simulink model "posture_regulation"  (R2022b)
settings: Solver=VariableStepAuto  StartTime=0.0  StopTime=20  RelTol=1e-3
model workspace (MAT data in the model file):
  initial_conditions = [0 0 0]
values from neighbouring files (symbols this model uses):
  initial_conditions_trans = state_transformation([0,0,0], initial_conditions)    [init.m]
settings Model: Creator=dipietrant  LastModifiedBy=Edp
settings SolverCC: AlgebraicLoopSolver=TrustRegion
settings DebuggingCC: UnconnectedInputMsg=warning  UnconnectedOutputMsg=warning  UnconnectedLineMsg=warning  SFMachineParentedDataDiag=warning
settings ModelReferenceCC: EnableRefExpFcnMdlSchedulingChecks=on
settings RTWCC: DLArmComputeVersion=19.05

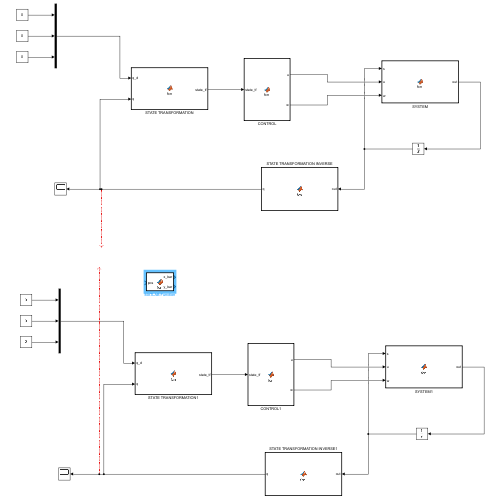
[thumbnail: Simulink's stored preview of the top-level diagram]
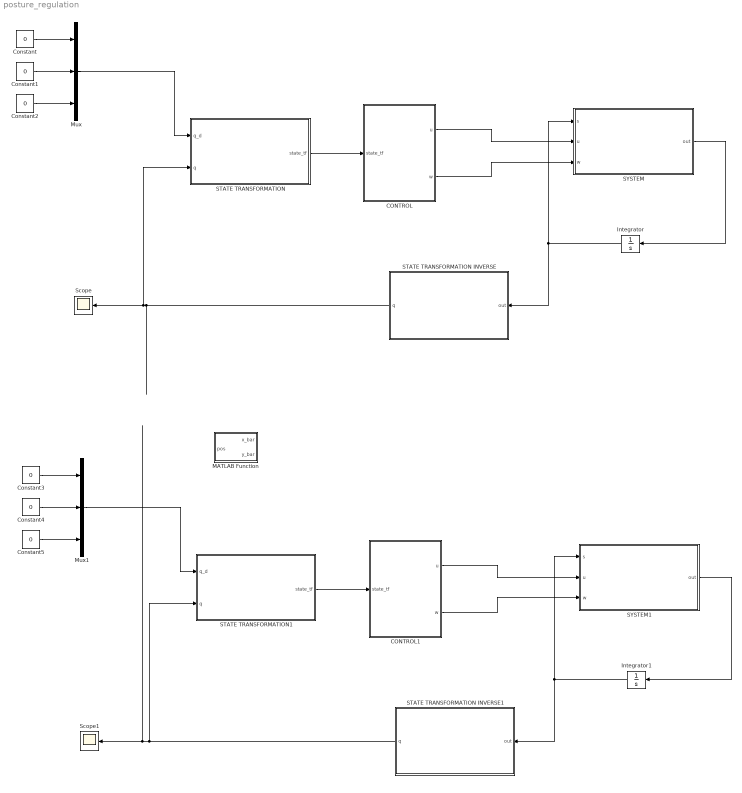
== system posture_regulation ==
  CONTROL : MATLAB Function  TreatAsAtomicUnit=on
  CONTROL1 : MATLAB Function  TreatAsAtomicUnit=on
  Constant{,1..5} (6 alike) : Constant  Value=0
  Integrator : Integrator  InitialCondition=initial_conditions_trans
  Integrator1 : Integrator  InitialCondition=initial_conditions_trans
  MATLAB Function : MATLAB Function  TreatAsAtomicUnit=on
  Mux : Mux  Inputs=3
  Mux1 : Mux  Inputs=3
  STATE TRANSFORMATION : MATLAB Function  TreatAsAtomicUnit=on
  STATE TRANSFORMATION INVERSE : MATLAB Function  TreatAsAtomicUnit=on
  STATE TRANSFORMATION INVERSE1 : MATLAB Function  TreatAsAtomicUnit=on
  STATE TRANSFORMATION1 : MATLAB Function  TreatAsAtomicUnit=on
  SYSTEM : MATLAB Function  TreatAsAtomicUnit=on
  SYSTEM1 : MATLAB Function  TreatAsAtomicUnit=on
  Scope : Scope
  Scope1 : Scope
  wires:
  SYSTEM/1(out) -> Integrator/1
  Integrator/1 -> SYSTEM/1(s), STATE TRANSFORMATION INVERSE/1(out)
  Constant/1 -> Mux/1
  Constant1/1 -> Mux/2
  Constant2/1 -> Mux/3
  Mux/1 -> STATE TRANSFORMATION/1(q_d)
  STATE TRANSFORMATION INVERSE/1(q) -> Scope/1, STATE TRANSFORMATION/2(q)
  CONTROL/1(u) -> SYSTEM/2(u)
  CONTROL/2(w) -> SYSTEM/3(w)
  STATE TRANSFORMATION/1(state_tf) -> CONTROL/1(state_tf)
  STATE TRANSFORMATION1/1(state_tf) -> CONTROL1/1(state_tf)
  CONTROL1/1(u) -> SYSTEM1/2(u)
  CONTROL1/2(w) -> SYSTEM1/3(w)
  Constant3/1 -> Mux1/1
  Integrator1/1 -> SYSTEM1/1(s), STATE TRANSFORMATION INVERSE1/1(out)
  Mux1/1 -> STATE TRANSFORMATION1/1(q_d)
  Constant5/1 -> Mux1/3
  STATE TRANSFORMATION INVERSE1/1(q) -> Scope1/1, STATE TRANSFORMATION1/2(q)
  SYSTEM1/1(out) -> Integrator1/1
  Constant4/1 -> Mux1/2

== matlab function posture_regulation/STATE TRANSFORMATION ==
  data: q_d input; state_tf output; q input
function state_tf = fcn(q_d, q)

x = q(1);
y = q(2);
theta = q(3);

rho = sqrt(x^2 + y^2);
gamma = atan2(y,x) + pi - theta;
delta = gamma + theta;

state_tf = [rho, gamma, delta];

== matlab function posture_regulation/CONTROL ==
  data: state_tf input; u output; w output
function [u, w]= fcn(state_tf)
k1 = 1;
k2 = 4;
k3 = 1;

rho = state_tf(1);
gamma = state_tf(2);
delta = state_tf(3);

u = k1 * cos(gamma);
w = k2 * gamma + k1*sin(gamma)*cos(gamma)/gamma*(gamma + k3*delta);

== matlab function posture_regulation/STATE TRANSFORMATION INVERSE ==
  data: out input; q output
function q = fcn(out)

rho = out(1);
gamma = out(2);
delta = out(3);

q = [0, 0, 0];
q(1) = -rho*cos(delta);
q(2) = -rho*sin(delta);
q(3) = delta - gamma;

== matlab function posture_regulation/SYSTEM ==
  data: s input; out output; u input; w input
function out = fcn(s, u, w)

rd = -s(1)*u*cos(s(2));
gd = u*sin(s(2)) - w;
dd = u*sin(s(2));

out = [rd, gd, dd];

== matlab function posture_regulation/CONTROL1 ==
  data: state_tf input; u output; w output
function [u, w]= fcn(state_tf)
k1 = 1;
k2 = 4;
k3 = 1;

rho = state_tf(1);
gamma = state_tf(2);
delta = state_tf(3);

u = k1 * cos(gamma);
w = k2 * gamma + k1*sin(gamma)*cos(gamma)/gamma*(gamma + k3*delta);

== matlab function posture_regulation/STATE TRANSFORMATION INVERSE1 ==
  data: out input; q output
function q = fcn(out)

rho = out(1);
gamma = out(2);
delta = out(3);

q = [0, 0, 0];
q(1) = -rho*cos(delta);
q(2) = -rho*sin(delta);
q(3) = delta - gamma;

== matlab function posture_regulation/STATE TRANSFORMATION1 ==
  data: q_d input; state_tf output; q input
function state_tf = fcn(q_d, q)

x = q(1);
y = q(2);
theta = q(3);

rho = sqrt(x^2 + y^2);
gamma = atan2(y,x) + pi - theta;
delta = gamma + theta;

state_tf = [rho, gamma, delta];

== matlab function posture_regulation/SYSTEM1 ==
  data: s input; out output; u input; w input
function out = fcn(s, u, w)

rd = -s(1)*u*cos(s(2));
gd = u*sin(s(2)) - w;
dd = u*sin(s(2));

out = [rd, gd, dd];

== matlab function posture_regulation/MATLAB Function ==
  data: pos input; x_bar output; y_bar output
function [x_bar, y_bar] = fcn(pos)

n = 0;
for i=1:3:length(pos)
    x_bar = x_bar + pos(i);
    y_bar = y_bar + pos(i+1);
    n = n + 1; 
end 

x_bar = x_bar / n;
y_bar = y_bar / n;
